simulink model "simulacion_seg_orden"  (R2021b)
settings: Solver=VariableStepAuto  StartTime=0.0  StopTime=10.0  RelTol=1e-3
settings Model: Creator=Alumno103  LastModifiedBy=Alumno103

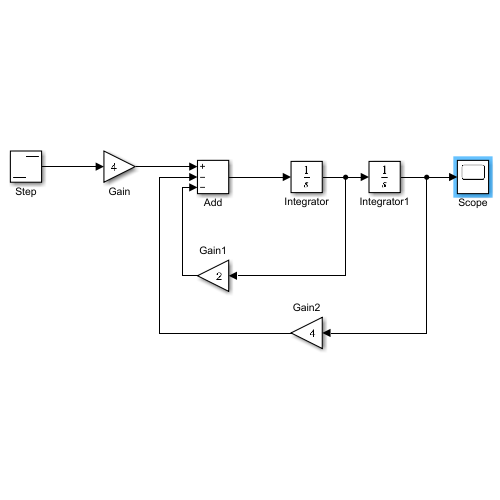
[thumbnail: Simulink's stored preview of the top-level diagram]
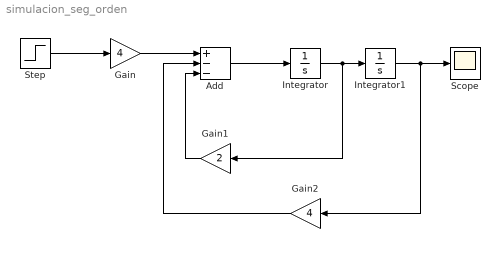
== system simulacion_seg_orden ==
  Add : Sum  Inputs=+--
  Gain : Gain  Gain=4
  Gain1 : Gain  Gain=2
  Gain2 : Gain  Gain=4
  Integrator : Integrator
  Integrator1 : Integrator
  Scope : Scope
  Step : Step  Time=0  SampleTime=0
  wires:
  Step/1 -> Gain/1
  Gain/1 -> Add/1
  Add/1 -> Integrator/1
  Gain1/1 -> Add/3
  Integrator/1 -> Gain1/1, Integrator1/1
  Integrator1/1 -> Gain2/1, Scope/1
  Gain2/1 -> Add/2
